simulink model "AM_DSB_TC_TX"  (R2024b)
settings: Solver=VariableStepAuto  StartTime=0.0  StopTime=inf  RelTol=1e-3
undefined symbols (not defined in the file): Fs, ip, usb
libraries: dspsrcs4 x3, dspmlti4 x2, plutoradiolib x1, dspvision x1
settings Model: Creator=javier.alonsov  LastModifiedBy=javit

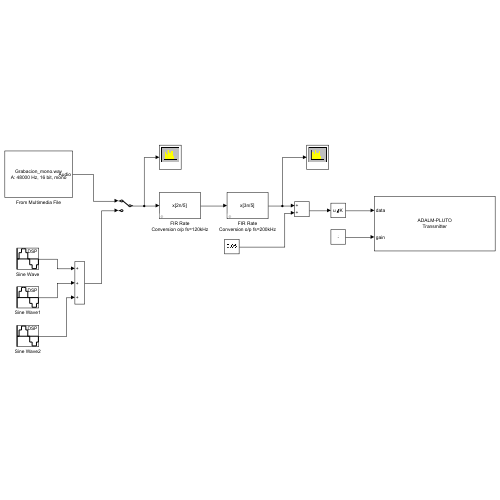
[thumbnail: Simulink's stored preview of the top-level diagram]
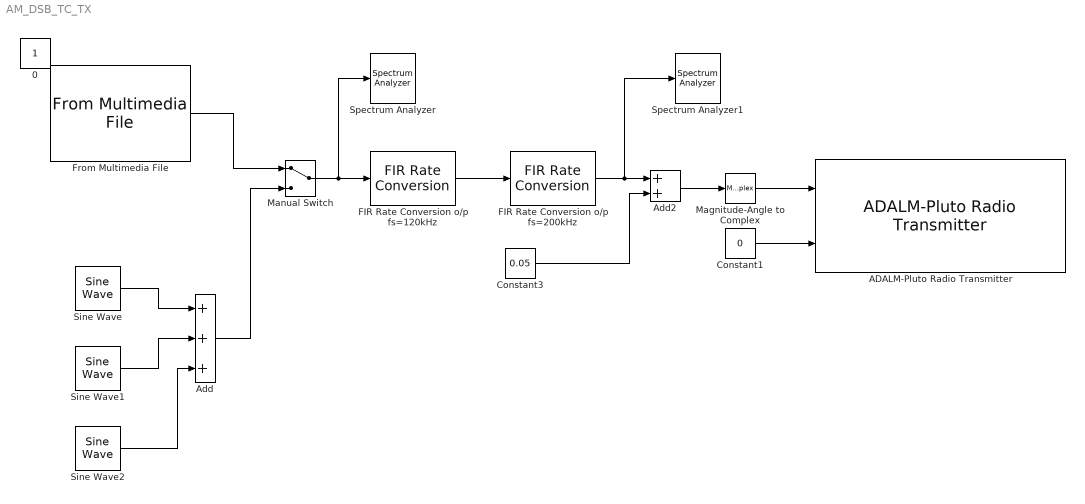
== system AM_DSB_TC_TX ==
  ADALM-Pluto Radio Transmitter : plutoradiolib/ADALM-Pluto Radio Transmitter  RadioID=usb:0  uri=ip:10.0.0.200  CenterFrequencySource=Dialog  CenterFrequency=433.9e6  GainSource=Input Port  Gain=-3  ChannelMapping=1  BasebandSampleRate=200e3  UnderflowOutputPort=off  ShowAdvancedProperties=off  UseCustomFilter=off  filtPathRates=[737280000 11520000 3840000 1920000 960000 240000]  filtCoefficients=[-192 82 85 -215 228 -102 -110 290 -318 145 160 -426 471 -215 -238 633 -697 318 349 -923 1009 -457 -498 1309 -1423 640 693 -1812 1959 -876 -945 2458 -2647 1180 1268 -3290 3534 -1572 -1688 4375 -4698 2091 2247 -5836 6284 -2807 -3031 7918 -8588 3870 4225 -11182 12324 -5662 -6330 17255 -19735 9507 11312 -33568 43355 -25227 -42139 305542 305542 -42139 -25227 43355 -33568 11312 9507 -19735 17255 -6330 -5662 12324 -11182 4225 3870 -8588 7918 -3031 -2807 6284 -5836 2247 2091 -4698 4375 -1688 -1572 3534 -3290 1268 1180 -2647 2458 -945 -876 1959 -1812 693 640 -1423 1309 -498 -457 1009 -923 349 318 -697 633 -238 -215 471 -426 160 145 -318 290 -110 -102 228 -215 85 82 -192]  filtCoefficientSize=128  filtDecimInterpFactor=4  filtGain=-12  filtRFBandwidth=18000000  filterConfigStruct=struct()  DataSourceSelect=Input Port  DDSTone1Freq=5e3  DDSTone2Freq=10e3  DDSTone1Scale=0.5  DDSTone2Scale=0.25  DataTimeout=Inf  FrequencyCorrection=0  ENSMPinControlMode=None  BISTLoopbackMode=Disabled  BISTToneInject=Disabled  BISTSignalGen=PRBS  BISTToneFreq=Fs/32  BISTToneLevel=0
  Add : Sum  Inputs=+++
  Add2 : Sum
  Constant1 : Constant  Value=0
  Constant3 : Constant  Value=0.05
  FIR Rate Conversion o/p fs=120kHz : dspmlti4/FIR Rate Conversion  FilterSource=Dialog parameters  L=5  h=firpm(50,[0 15e3 24e3 240e3/2]/(240e3/2),[1 1 0 0], [1 1],20)  M=2  FilterObject=FRC  rateMode=Enforce single-rate processing  AllowArbitraryInputLength=off  roundingMode=Floor  overflowMode=off  firstCoeffDataTypeStr=Inherit: Same word length as input  firstCoeffMin=[]  firstCoeffMax=[]  firstCoeffLastDataTypeStr=Inherit: Same word length as input  outputDataTypeStr=Inherit: Same as accumulator  outputMin=[]  outputMax=[]  outputLastDataTypeStr=Inherit: Same as accumulator
  FIR Rate Conversion o/p fs=200kHz : dspmlti4/FIR Rate Conversion  FilterSource=Dialog parameters  L=5  h=firpm(50,[0 15e3 30e3 600e3/2]/(600e3/2),[1 1 0 0], [1 1],20)  M=3  FilterObject=FRC  rateMode=Enforce single-rate processing  AllowArbitraryInputLength=off  roundingMode=Floor  overflowMode=off  firstCoeffDataTypeStr=Inherit: Same word length as input  firstCoeffMin=[]  firstCoeffMax=[]  firstCoeffLastDataTypeStr=Inherit: Same word length as input  outputDataTypeStr=Inherit: Same as accumulator  outputMin=[]  outputMax=[]  outputLastDataTypeStr=Inherit: Same as accumulator
  From Multimedia File : dspvision/From Multimedia File  inputFilename=C:\Users\javit\Documents\Curso25_26\Docencia\GET\SISCOM\LAB\SDR_3_DesmodAMNoCoherent\Grabacion_mono.wav  readRange=[1 Inf]  loop=on  numPlays=inf  outputStreams=Audio only  videoDataType=single  audioDataType=single  inheritSampleTime=on  userDefinedSampleTime=1/30  noAudioOutput=off  isIntensityVideo=off  fourcc=RGB  colorVideoFormat=One multidimensional signal  outputEOF=off  dataOrg=Column-major  audioFrameSize=600  computeAudioFrameSize=off  outSamplingMode=Sample based
      settings: LibrarySourceBlock=dspsrcs4/From Multimedia File
  Magnitude-Angle to Complex : MagnitudeAngleToComplex  Input=Magnitude
  Manual Switch : ManualSwitch
  Sine Wave : dspsrcs4/Sine Wave  Amplitude=0.025  Frequency=1e3  Phase=0  SampleMode=Discrete  OutComplex=Real  CompMethod=Trigonometric fcn  TableSize=Speed  SampleTime=1/48e3  SamplesPerFrame=600  ResetState=Restart at time zero  OutputFrames=off  dataType=double  wordLen=16  udDataType=sfix(16)  fracBitsMode=Best precision  numFracBits=15  OutDataTypeStr=double  LastOutDataTypeStr=double
  Sine Wave1 : dspsrcs4/Sine Wave  Amplitude=0.025  Frequency=5e3  Phase=0  SampleMode=Discrete  OutComplex=Real  CompMethod=Trigonometric fcn  TableSize=Speed  SampleTime=1/48e3  SamplesPerFrame=600  ResetState=Restart at time zero  OutputFrames=off  dataType=double  wordLen=16  udDataType=sfix(16)  fracBitsMode=Best precision  numFracBits=15  OutDataTypeStr=double  LastOutDataTypeStr=double
  Sine Wave2 : dspsrcs4/Sine Wave  Amplitude=0.025  Frequency=8e3  Phase=0  SampleMode=Discrete  OutComplex=Real  CompMethod=Trigonometric fcn  TableSize=Speed  SampleTime=1/48e3  SamplesPerFrame=600  ResetState=Restart at time zero  OutputFrames=off  dataType=double  wordLen=16  udDataType=sfix(16)  fracBitsMode=Best precision  numFracBits=15  OutDataTypeStr=double  LastOutDataTypeStr=double
  Spectrum Analyzer : SpectrumAnalyzer  WindowPosition=[4233.000000,-463.000000,800.000000,500.000000,]  ScopeFrameLocation=window  SpectrumType=RMS  Method=Welch  AxesScaling=Manual  FrequencyResolutionMethod=Window length  WindowInvariantSamplesPerUpdate=on  SpectrumUnits=Vrms  ReferenceLoad=50  YLimits=[-2 2]
  Spectrum Analyzer1 : SpectrumAnalyzer  WindowPosition=[3153.000000,-459.000000,800.000000,500.000000,]  ScopeFrameLocation=window  SpectrumType=RMS  Method=Welch  AxesScaling=Manual  FrequencyResolutionMethod=Window length  WindowInvariantSamplesPerUpdate=on  SpectrumUnits=Vrms  ReferenceLoad=50  YLimits=[-0.06436269501271685,0.10959955854771326]
  0 : Constant  IOType=siggen
  wires:
  FIR Rate Conversion o/p fs=120kHz/1 -> FIR Rate Conversion o/p fs=200kHz/1
  Manual Switch/1 -> Spectrum Analyzer/1, FIR Rate Conversion o/p fs=120kHz/1
  From Multimedia File/1 -> Manual Switch/1
  Sine Wave/1 -> Add/1
  Sine Wave1/1 -> Add/2
  Sine Wave2/1 -> Add/3
  Add/1 -> Manual Switch/2
  FIR Rate Conversion o/p fs=200kHz/1 -> Spectrum Analyzer1/1, Add2/1
  Constant3/1 -> Add2/2
  Add2/1 -> Magnitude-Angle to Complex/1
  Magnitude-Angle to Complex/1 -> ADALM-Pluto Radio Transmitter/1
  Constant1/1 -> ADALM-Pluto Radio Transmitter/2
